simulink model "CE3_3_sim"  (R2019b)
settings: Solver=VariableStepAuto  StartTime=0.0  StopTime=500  RelTol=1e-3
values from neighbouring files (symbols this model uses):
  A1 = [1 -1.87725934651 0.340802185942 0.77661620255 -0.0146133638787 -0.228390117055 0.00387237190516]    [CE3_3.mat]
  A2 = [1 -1.67710055601 0.25148798104 0.589524996758 -0.119638880328 0.109659430706 -0.148420178812]    [CE3_3.mat]
  A3 = [1 -1.62662080159 0.19228858332 0.440533319966 0.161606022913 0.00463579188745 -0.166992521201]    [CE3_3.mat]
  B1 = [0 0.0147825272812 0.0034510072183 -0.0171453222772 -0.0138159676186 0.00488453572954 0.00886970257631]    [CE3_3.mat]
  B2 = [0 0.0145960982534 0.00573848925416 -0.0119560959313 -0.010558728223 0.00173493544932 0.00620559610866]    [CE3_3.mat]
  B3 = [0 0.0148241435876 0.00522838271059 -0.0112846379366 -0.0107140318229 0.00279863501769 0.00506613371561]    [CE3_3.mat]
  Ts = 0.02    [CE3_3.mat]    (also in id_data.mat)
undefined symbols (not defined in the file or in its folder): D1, D2, D3, N1, N2, N3
libraries: cstblocks x3
settings Model: Creator=Silvio  LastModifiedBy=Silvio
settings DataIOCC: ReturnWorkspaceOutputs=off

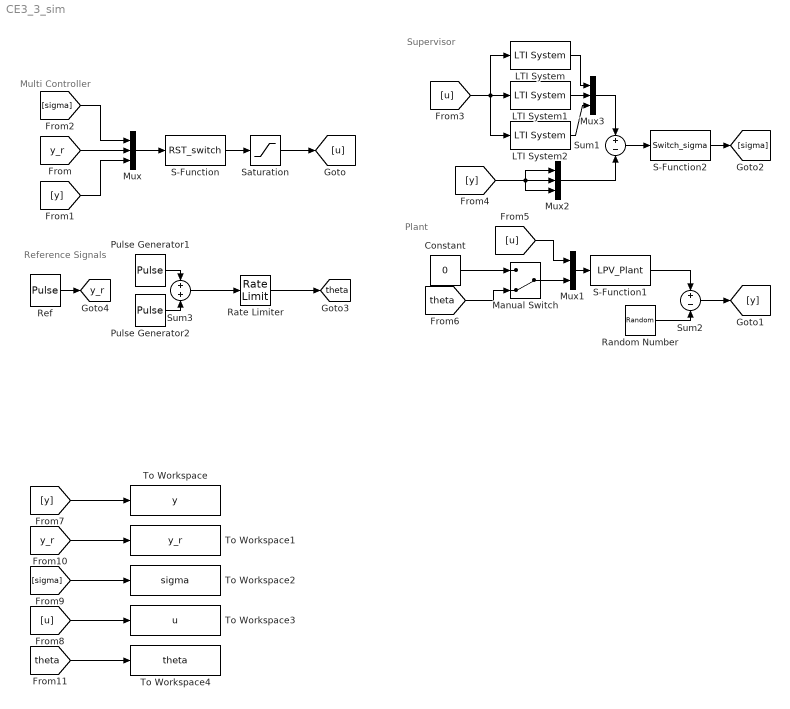
== system CE3_3_sim ==
  note: Supervisor
  note: Plant
  note: Multi Controller
  note: Reference Signals
  Constant : Constant  Value=0
  LTI System : cstblocks/LTI System  sys=tf(B1,A1,Ts)  IC=[]
  LTI System1 : cstblocks/LTI System  sys=tf(B2,A2,Ts)  IC=[]
  LTI System2 : cstblocks/LTI System  sys=tf(B3,A3,Ts)  IC=[]
  Manual Switch : ManualSwitch  CurrentSetting=0
  Mux : Mux  Inputs=3
  Mux1 : Mux  Inputs=2
  Mux2 : Mux  Inputs=3
  Mux3 : Mux  Inputs=3
  Pulse Generator1 : DiscretePulseGenerator  PulseType=Time based  Period=200  PulseWidth=50
  Pulse Generator2 : DiscretePulseGenerator  PulseType=Time based  Amplitude=-1  Period=200  PulseWidth=50  PhaseDelay=50
  Random Number : RandomNumber  Variance=0.00001  SampleTime=Ts
  Rate Limiter : RateLimiter  RisingSlewLimit=0.05  FallingSlewLimit=-0.05  SampleTimeMode=inherited
  Ref : DiscretePulseGenerator  PulseType=Time based  Amplitude=0.5  Period=10  PulseWidth=50
  S-Function : S-Function  FunctionName=RST_switch  Parameters=N1,D1,N2,D2,N3,D3,Ts  SFunctionDeploymentMode=off  EnableBusSupport=off
  S-Function1 : S-Function  FunctionName=LPV_Plant  Parameters=A1,B1,A2,B2,A3,B3,Ts  SFunctionDeploymentMode=off  EnableBusSupport=off
  S-Function2 : S-Function  FunctionName=Switch_sigma  Parameters=alpha, lambda, DT, Ts  SFunctionDeploymentMode=off  EnableBusSupport=off
  Saturation : Saturate  UpperLimit=5  LowerLimit=-5
  Sum1 : Sum  Inputs=+-
  Sum2 : Sum  Inputs=+-
  Sum3 : Sum
  To Workspace : ToWorkspace  VariableName=y  SaveFormat=Timeseries  SampleTime=-1
  To Workspace1 : ToWorkspace  VariableName=y_r  SaveFormat=Timeseries  SampleTime=-1
  To Workspace2 : ToWorkspace  VariableName=sigma  SaveFormat=Timeseries  SampleTime=-1
  To Workspace3 : ToWorkspace  VariableName=u  SaveFormat=Timeseries  SampleTime=-1
      settings: Save2DSignal=2-D array (concatenate along first dimension)
  To Workspace4 : ToWorkspace  VariableName=theta  SaveFormat=Timeseries  SampleTime=-1
      settings: Save2DSignal=2-D array (concatenate along first dimension)
  tag scope: theta=global, y_r=global
  wires:
  Ref/1 -> [y_r]
  Pulse Generator2/1 -> Sum3/2
  Rate Limiter/1 -> [theta]
  Pulse Generator1/1 -> Sum3/1
  Sum3/1 -> Rate Limiter/1
  Mux/1 -> S-Function/1
  [y] -> Mux/3
  [sigma] -> Mux/1
  [y_r] -> Mux/2
  S-Function2/1 -> [sigma]
  [u] -> Mux1/1
  Mux1/1 -> S-Function1/1
  [y] -> Mux2/1, Mux2/3, Mux2/2
  Mux2/1 -> Sum1/2
  Mux3/1 -> Sum1/1
  Sum1/1 -> S-Function2/1
  [u] -> LTI System2/1, LTI System1/1, LTI System/1
  LTI System2/1 -> Mux3/3
  LTI System1/1 -> Mux3/2
  LTI System/1 -> Mux3/1
  Saturation/1 -> [u]
  S-Function/1 -> Saturation/1
  Constant/1 -> Manual Switch/1
  [theta] -> Manual Switch/2
  Manual Switch/1 -> Mux1/2
  [y] -> To Workspace/1
  [y_r] -> To Workspace1/1
  [sigma] -> To Workspace2/1
  [u] -> To Workspace3/1
  [theta] -> To Workspace4/1
  S-Function1/1 -> Sum2/1
  Sum2/1 -> [y]
  Random Number/1 -> Sum2/2
